simulink model "AEB_sliding_mode_Control"  (R2021b)
settings: Solver=ode4  StartTime=0.0  StopTime=18  FixedStep=simtime  RelTol=1e-3
InitFcn:
  | clear all
  | 
  | % These are the starting values
  | initial_stopping_distance = 350; % set the stopping distance in m (6.368 and 11 is max deccel -9.5)
  | initial_velocity = 37.77; % set the initial velocity in m/s
  | road_grade = 0; %set road grade in degrees
  | sampletime = 0.01; %set the sample time of the controller
  | Ts = sampletime;
  | simtime = sampletime; %simulation set
  | 
  | initialdeccelcalc = -(initial_velocity^2)/(2*initial_stopping_distance);
undefined symbols (not defined in the file): magnitude
libraries: simulink x2, sim3dlib x2, vdynlib x2, sim3dprobsensorlib x1, dspvision x1, autolibshared x1
settings Model: Creator=Tanmay Panchal  LastModifiedBy=tapan
settings SolverCC: AlgebraicLoopSolver=TrustRegion
settings DebuggingCC: SFMachineParentedDataDiag=warning

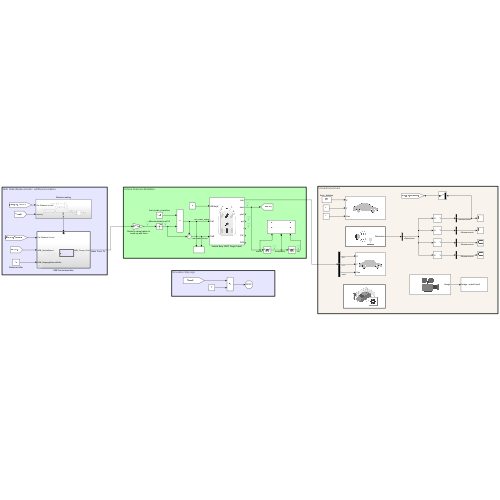
[thumbnail: Simulink's stored preview of the top-level diagram]
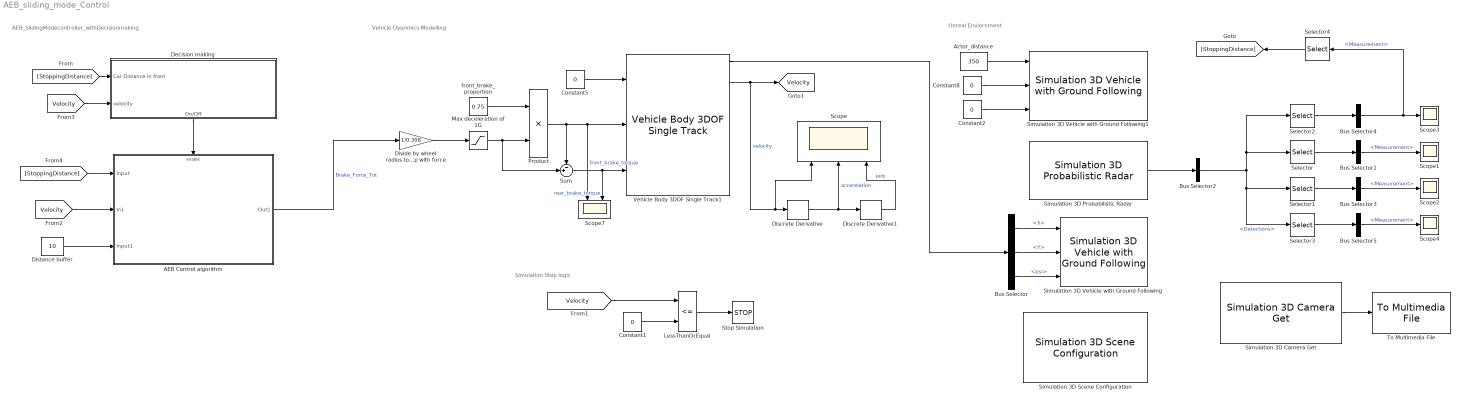
== system AEB_sliding_mode_Control ==
  note: AEB_SlidingModecontroller_withDecisionmaking
  note: Vehicle Dyanmics Modelling
  note: Unreal Enviornment
  note: Simulation Stop logic
  AEB Control algorithm : Subsystem  AncestorBlock=autonomous_emergency_braking/Enabled Subsystem  TreatAsAtomicUnit=on
  Actor_distance : Constant  Value=350
  Bus Selector : BusSelector  OutputSignals=InertFrm.Cg.Disp.X,InertFrm.Cg.Disp.Y,InertFrm.Cg.Ang.psi
  Bus Selector{1,3..5} (4 alike) : BusSelector  OutputSignals=Measurement
  Bus Selector2 : BusSelector  OutputSignals=Detections
  Constant{1..2,5,8} (4 alike) : Constant  Value=0
  Decision making : Subsystem
      settings: PortSchema="{\"entries\":[{\"content\":{\"sides\":[{\"content\":{\"connectorIds\":[\"In1\",\"In2\"]},\"type\":\"ConnectorPlacement.EquallySpacedRectSide\",\"uuid\":\"07d6ad26-48ba-4c38-b484-67a208300176\"},{\"content\":{\"connectorIds\":[],\"side\":\"RIGHT\"},\"type\":\"ConnectorPlacement.EquallySpacedRectSide\",\"uuid\":\"bb97d993-8e0c-453d-bb06-d9e692861d0d\"},{\"content\":{\"connectorIds\":[],\"side\":\"TOP\"},\"type\":\"ConnectorPlacement.EquallySpacedRectSide\",\"uuid\":\"8aa86946-bb58-4dea-97e3-c73328440966\"},{\"content\":{\"connectorIds\":[\"Out1\"],\"side\":\"BOTTOM\"},\"type\":\"ConnectorPlacement.EquallySpacedRectSide\",\"uuid\":\"cee6b2ec-0c05-4422-9818-dbb41960cecd\"}]},\"type\":\"ConnectorPlacement.EquallySpacedConnector\",\"uuid\":\"33f67331-c5e1-42c8-9d75-589712a9155e\"}],\"packageUris\":[\"http://schema.mathworks.com/mf0/Connector/R2020b\"],\"version\":\"1.0\"}"
  Discrete Derivative : simulink/Discrete/Discrete Derivative  gainval=1.0  ICPrevScaledInput=initial_velocity/sampletime  OutMin=[]  OutMax=[]  OutDataType=fixdt(1, 16)  OutScaling=2^-10  DoSatur=off
  Discrete Derivative1 : simulink/Discrete/Discrete Derivative  gainval=1.0  ICPrevScaledInput=0.0  OutMin=[]  OutMax=[]  OutDataType=fixdt(1, 16)  OutScaling=2^-10  DoSatur=off
  Distance buffer : Constant  Value=10
  Divide by wheel radius to come up with force : Gain  Gain=1/0.308
  LessThanOrEqual : RelationalOperator  Operator=<=  OutDataTypeStr=boolean  RndMeth=Simplest
  Max deceleration of 1G : Saturate  UpperLimit=0  LowerLimit=-1605*10
  Product : Product
  Scope : Scope  NumInputPorts=3
  Scope{1..4} (4 alike) : Scope
  Scope7 : Scope  NumInputPorts=2
  Selector : Selector  InputPortWidth=10  IndexOptions=Index vector (dialog)  Indices=[3]  OutputSizes=1
  Selector1 : Selector  InputPortWidth=10  IndexOptions=Index vector (dialog)  Indices=[5]  OutputSizes=1
  Selector2 : Selector  InputPortWidth=10  IndexOptions=Index vector (dialog)  Indices=[1]  OutputSizes=1
  Selector3 : Selector  InputPortWidth=10  IndexOptions=Index vector (dialog)  Indices=[7]  OutputSizes=1
  Selector4 : Selector  InputPortWidth=3  IndexOptions=Index vector (dialog)  Indices=[1]  OutputSizes=1
  Simulation 3D Camera Get : sim3dlib/Simulation 3D Camera Get  Priority=1  sensorTag=Sim3dSensor3  sensorId=3  sensorName=Sim3dSensor3  vehTagList={'EGOVehicle';'Scene Origin';'Stray'}  vehTag=EGOVehicle  mountLoc=Rearview mirror  offsetFlag=off  tmountOffset=[0, 0, 0]  rmountOffset=[0, 0, 0]  HorizontalResolution=1280  VerticalResolution=720  HorizontalFOV=60  SampleTime=-1  mountPoint=[0.389999985694885 0 1.53999996185303]  mountOrientation=[0 0 0]  aMode=2  ID=3
      settings: SourceProductBaseCode=AE,DR,UV,VE
  Simulation 3D Probabilistic Radar : sim3dprobsensorlib/Simulation 3D Probabilistic Radar  Priority=1  sensorTag=Sim3dSensor1  sensorId=1  sensorName=Sim3dSensor1  vehTagList={'EGOVehicle';'Scene Origin';'Stray'}  vehTag=EGOVehicle  mountLoc=Origin  offsetFlag=off  tmountOffset=[0, 0, 0]  rmountOffset=[0, 0, 0]  AzimuthResolution=4  ElevationResolution=10  RangeResolution=2.5  RangeRateResolution=0.5  AzimuthBiasFraction=0.1  ElevationBiasFraction=0.1  RangeBiasFraction=0.05  RangeRateBiasFraction=0.05  FieldOfView=[ 20, 5 ]  DetectionRange=[ 1, 300 ]  RangeRateLimits=[ -100, 100 ]  DetectionProbability=0.9  FalseAlarmRate=1e-6  ReferenceRange=1000  ReferenceRCS=0  HasElevation=on  HasRangeRate=off  HasNoise=off  HasFalseAlarms=off  InitialSeedSource=Repeatable  InitialSeed=0  MaxNumDetections=10  DetectionCoordinates=Sensor Cartesian  SpecifyOutputBusName=off  BusName=BusSimulation3DRadarTruthSensor  SampleTime=-1  mountPoint=[0 0 0]  mountOrientation=[0 0 0]  aMode=3  ID=1
      settings: SourceProductBaseCode=AE,DR,UV,VE
  Simulation 3D Scene Configuration : sim3dlib/Simulation 3D Scene Configuration  Priority=0  ProjectFormat_internal=Default Scenes  ProjectFormat=Default Scenes  SceneDesc=Straight road  ProjectName=C:\Program Files\MATLAB\R2021b\toolbox\shared\sim3d_projects\automotive_project\UE4\WindowsNoEditor\VehicleSimulation.exe  ScenePath=/Game/Maps/HwStrght  vehTagList={'EGOVehicle';'Scene Origin';'Stray'}  vehTag=EGOVehicle  OpVisEn=off  Ts=0.01  EnableWindow=off  EnableWeather=off  SunAltitude=40.0  SunAzimuth=90  clouds=10  wind=1  fog=0  rain=0  sensorTag=MainCamera1  sensorId=1  sensorName=MainCamera1  mountLoc=Origin  offsetFlag=off  tmountOffset=[0, 0, 0]  rmountOffset=[0, 0, 0]  HorizontalResolution=1280  VerticalResolution=720  HorizontalFOV=60  mountPoint=[0 0 0]  mountOrientation=[0 0 0]  aMode=3  ID=1
      settings: SourceProductBaseCode=AE,DR,UV,VE
  Simulation 3D Vehicle with Ground Following : vdynlib/Vehicle Scenarios/Sim3D/Sim3D Vehicle/Components/Simulation 3D Vehicle with Ground Following  Priority=-1  PassVehMesh=Sport utility vehicle  PassVehMesh_Internal=Sport utility vehicle  MeshPath=/MathWorksSimulation/Vehicles/Muscle/Meshes/SK_MuscleCar.SK_MuscleCar  TrackWidth=1.9  WheelBase=3  WheelRadius=0.35  VehColor=Silver  VehColor_Internal=Silver  InitialPos=[0, 0, 0]  InitialRot=[0, 0, 0]  ActorName=EGOVehicle  VehLightsControl=off  HeadlightColor=[ 1, 1, 1 ]  HighBeamIntensity=100000  LowBeamIntensity=60000  HighBeamConeAngle=1.22  LowBeamConeAngle=1.22  LeftHeadlightOrientation=[ 0, 0 ]  RightHeadlightOrientation=[ 0, 0 ]  BrakelightIntensity=200  ReverselightIntensity=500  SignallightIntensity=500  SignallightPeriod=1  SignalPulseWidth=50  SampleTime=-1  ActorType=SimulinkVehicle  ID=C  aMode=2  ActorTag=EGOVehicle  CoordinateScheme=SAE
      settings: SourceProductBaseCode=VE
  Simulation 3D Vehicle with Ground Following1 : vdynlib/Vehicle Scenarios/Sim3D/Sim3D Vehicle/Components/Simulation 3D Vehicle with Ground Following  Priority=-1  PassVehMesh=Muscle car  PassVehMesh_Internal=Muscle car  MeshPath=/MathWorksSimulation/Vehicles/Muscle/Meshes/SK_MuscleCar.SK_MuscleCar  TrackWidth=1.9  WheelBase=3  WheelRadius=0.35  VehColor=Yellow  VehColor_Internal=Yellow  InitialPos=[0, 5, 0]  InitialRot=[0, 0, 0]  ActorName=Stray  VehLightsControl=off  HeadlightColor=[ 1, 1, 1 ]  HighBeamIntensity=100000  LowBeamIntensity=60000  HighBeamConeAngle=1.22  LowBeamConeAngle=1.22  LeftHeadlightOrientation=[ 0, 0 ]  RightHeadlightOrientation=[ 0, 0 ]  BrakelightIntensity=200  ReverselightIntensity=500  SignallightIntensity=500  SignallightPeriod=1  SignalPulseWidth=50  SampleTime=-1  ActorType=SimulinkVehicle  ID=C  aMode=2  ActorTag=Stray  CoordinateScheme=SAE
      settings: SourceProductBaseCode=VE
  Stop Simulation : Stop
  Sum : Sum  Inputs=-+|
  To Multimedia File : dspvision/To Multimedia File  outputFilename=C:\Users\tapan\Desktop\output2.mp4  streamSelection=Video only  videoCompressor=None (uncompressed)  audioCompressor=None (uncompressed)  imagePorts=One multidimensional signal  fileType=MPEG4  audioDatatype=Determine from input data type  fourcc=RGB  videoQuality=75  mj2000CompFactor=10
  Vehicle Body 3DOF Single Track1 : autolibshared/Vehicle Body 3DOF Single Track  trackMode=Single (bicycle)  inputMode=External longitudinal forces  frontSteerMode=on  rearSteerMode=off  windMode=off  muMode=off  extFMode=off  extMMode=off  htchFMode=off  htchMMode=off  extXo=off  extpsio=off  extxdoto=off  extro=off  extYo=off  extTamb=off  extydoto=off  aMode=2  NF=2  NR=2  m=1625  a=1.135  b=1.465  h=0.509  dh=1  hh=0.2  X_o=0  xdot_o=initial_velocity  CalphaMode=off  sigmaMode=on  d=0  hl=0  w=[1.4,1.4]  Cy_f=12e3  Cy_r=11e3  sigma_f=.1  sigma_r=.1  alpha_f_brk=[-.1 .1]  Cy_f_data=[-9e3 9e3]  alpha_r_brk=[-.1 .1]  Cy_r_data=[-9e3 9e3]  Y_o=0  ydot_o=0  Izz=2045  psi_o=0  r_o=0  Af=2  Cd=.3  Cl=.1  Cpm=.1  beta_w=[0:0.01:0.3]  Cs=[0:0.03:0.9]  Cym=[0:0.01:0.3]  Pabs=101325  Tair=273  g=9.81  mu=1  xdot_tol=.01  Fznom=5000  Fxtire_sat=7e4  Fytire_sat=7e4  longOff=0  latOff=0  vertOff=0  wrapAng=off
      settings: SourceProductBaseCode=PW,DR,MT,UV,VE
  front_brake_proportion : Constant  Value=0.75
  tag scope: Velocity=global
  wires:
  Discrete Derivative/1 -> Discrete Derivative1/1, Scope/2  "accerelation"
  Vehicle Body 3DOF Single Track1/2 -> Scope/1, Discrete Derivative/1, [Velocity]  "velocity"
  Discrete Derivative1/1 -> Scope/3  "jerk"
  LessThanOrEqual/1 -> Stop Simulation/1
  [Velocity] -> LessThanOrEqual/1
  Constant5/1 -> Vehicle Body 3DOF Single Track1/1
  Divide by wheel radius to come up with force/1 -> Max deceleration of 1G/1
  Max deceleration of 1G/1 -> Sum/2, Product/2
  Sum/1 -> Vehicle Body 3DOF Single Track1/3, Scope7/2  "rear_brake_torque"
  front_brake_proportion/1 -> Product/1
  Product/1 -> Scope7/1, Vehicle Body 3DOF Single Track1/2, Sum/1  "front_brake_torque"
  Bus Selector/2 -> Simulation 3D Vehicle with Ground Following/2  "<Y>"
  Bus Selector/1 -> Simulation 3D Vehicle with Ground Following/1  "<X>"
  Bus Selector/3 -> Simulation 3D Vehicle with Ground Following/3  "<psi>"
  Vehicle Body 3DOF Single Track1/1 -> Bus Selector/1
  Constant2/1 -> Simulation 3D Vehicle with Ground Following1/3
  Constant8/1 -> Simulation 3D Vehicle with Ground Following1/2
  Actor_distance/1 -> Simulation 3D Vehicle with Ground Following1/1
  Simulation 3D Probabilistic Radar/1 -> Bus Selector2/1
  Bus Selector2/1 -> Selector/1, Selector2/1, Selector3/1, Selector1/1  "<Detections>"
  Selector/1 -> Bus Selector1/1
  Bus Selector1/1 -> Scope1/1  "<Measurement>"
  Bus Selector3/1 -> Scope2/1  "<Measurement>"
  Selector1/1 -> Bus Selector3/1
  Selector2/1 -> Bus Selector4/1
  Bus Selector4/1 -> Selector4/1, Scope3/1  "<Measurement>"
  Bus Selector5/1 -> Scope4/1  "<Measurement>"
  Selector3/1 -> Bus Selector5/1
  Distance buffer/1 -> AEB Control algorithm/3(Input1)
  Decision making/1(On/Off) -> AEB Control algorithm/Enable
  Simulation 3D Camera Get/1 -> To Multimedia File/1
  [Velocity] -> AEB Control algorithm/2(In1)
  [Velocity] -> Decision making/2(velocity)
  AEB Control algorithm/1(Out1) -> Divide by wheel radius to come up with force/1  "Brake_Force_Tot"
  Constant1/1 -> LessThanOrEqual/2
  Selector4/1 -> [StoppingDistance]
  [StoppingDistance] -> Decision making/1(Car Distance in front)
  [StoppingDistance] -> AEB Control algorithm/1(Input)

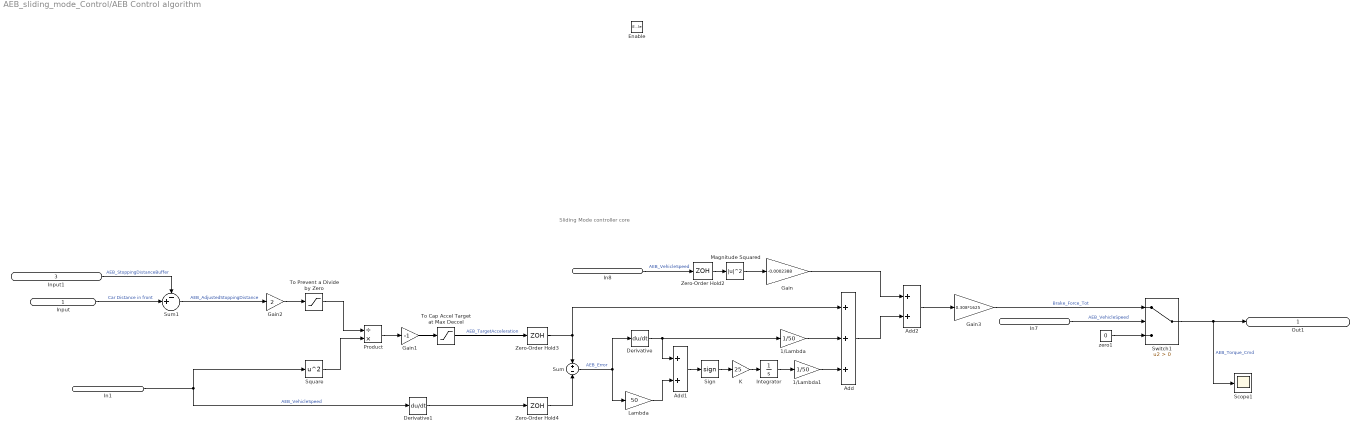
== system AEB_sliding_mode_Control/AEB Control algorithm ==
  note: Sliding Mode controller core
  Input : Inport
  In1 : Inport  Port=2
  Input1 : Inport  Port=3
  Enable : EnablePort
  1/Lambda : Gain  Gain=1/50
  1/Lambda1 : Gain  Gain=1/50
  Add : Sum  Inputs=+++
  Add1 : Sum
  Add2 : Sum
  Derivative : Derivative
  Derivative1 : Derivative
  Gain : Gain  Gain=-0.0002388
  Gain1 : Gain  Gain=-1
  Gain2 : Gain  Gain=2
  Gain3 : Gain  Gain=0.308*1625
  In7 : InportShadow  Port=2
  In8 : InportShadow  Port=2
  Integrator : Integrator
  K : Gain  Gain=25
  Lambda : Gain  Gain=50
  Magnitude Squared : Math  Operator=magnitude^2  SaturateOnIntegerOverflow=on
  Product : Product  Inputs=/*
  Scope1 : Scope
  Sign : Signum
  Square : Math  Operator=square  SaturateOnIntegerOverflow=on
  Sum : Sum  Inputs=+|-
  Sum1 : Sum  Inputs=-+|
  Switch1 : Switch  Criteria=u2 > Threshold
  To Cap Accel Target at Max Deccel : Saturate  UpperLimit=0  LowerLimit=-9.81
  To Prevent a Divide by Zero : Saturate  UpperLimit=inf  LowerLimit=0.001
  Zero-Order Hold2 : ZeroOrderHold  SampleTime=0.01
  Zero-Order Hold3 : ZeroOrderHold  SampleTime=0.01
  Zero-Order Hold4 : ZeroOrderHold  SampleTime=0.01
  zero1 : Constant  Value=0
  Out1 : Outport
  wires:
  In1/1 -> Derivative1/1, Square/1  "AEB_VehicleSpeed"
  Gain2/1 -> To Prevent a Divide by Zero/1
  To Cap Accel Target at Max Deccel/1 -> Zero-Order Hold3/1  "AEB_TargetAcceleration"
  Gain1/1 -> To Cap Accel Target at Max Deccel/1
  Sum1/1 -> Gain2/1  "AEB_AdjustedStoppingDistance"
  Input1/1 -> Sum1/1  "AEB_StoppingDistanceBuffer"
  Product/1 -> Gain1/1
  Square/1 -> Product/2
  To Prevent a Divide by Zero/1 -> Product/1
  Input/1 -> Sum1/2  "Car Distance in front"
  Sum/1 -> Derivative/1, Lambda/1  "AEB_Error"
  In7/1 -> Switch1/2  "AEB_VehicleSpeed"
  Gain3/1 -> Switch1/1  "Brake_Force_Tot"
  zero1/1 -> Switch1/3
  In8/1 -> Zero-Order Hold2/1  "AEB_VehicleSpeed"
  Magnitude Squared/1 -> Gain/1
  1/Lambda/1 -> Add/2
  Derivative/1 -> 1/Lambda/1, Add1/1
  1/Lambda1/1 -> Add/3
  Lambda/1 -> Add1/2
  Add1/1 -> Sign/1
  Integrator/1 -> 1/Lambda1/1
  K/1 -> Integrator/1
  Sign/1 -> K/1
  Add/1 -> Add2/2
  Zero-Order Hold3/1 -> Sum/1, Add/1
  Zero-Order Hold2/1 -> Magnitude Squared/1
  Switch1/1 -> Scope1/1, Out1/1  "AEB_Torque_Cmd"
  Add2/1 -> Gain3/1
  Zero-Order Hold4/1 -> Sum/2
  Gain/1 -> Add2/1
  Derivative1/1 -> Zero-Order Hold4/1

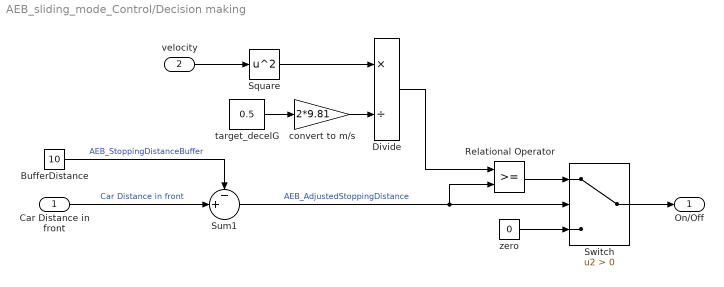
== system AEB_sliding_mode_Control/Decision making ==
  Car Distance in front : Inport
  velocity : Inport  Port=2
  BufferDistance : Constant  Value=10
  Divide : Product  Inputs=*/
  Relational Operator : RelationalOperator  OutDataTypeStr=boolean  RndMeth=Simplest
  Square : Math  Operator=square  SaturateOnIntegerOverflow=on
  Sum1 : Sum  Inputs=-+|
  Switch : Switch  Criteria=u2 > Threshold
  convert to m/s : Gain  Gain=2*9.81
  target_decelG : Constant  Value=0.5
  zero : Constant  Value=0
  On/Off : Outport
  wires:
  velocity/1 -> Square/1
  Square/1 -> Divide/1
  Divide/1 -> Relational Operator/1
  zero/1 -> Switch/3
  convert to m/s/1 -> Divide/2
  Relational Operator/1 -> Switch/1
  target_decelG/1 -> convert to m/s/1
  Switch/1 -> On/Off/1
  Car Distance in front/1 -> Sum1/2  "Car Distance in front"
  Sum1/1 -> Relational Operator/2, Switch/2  "AEB_AdjustedStoppingDistance"
  BufferDistance/1 -> Sum1/1  "AEB_StoppingDistanceBuffer"
